simulink model "Cruise_model"  (R2020a)
settings: Solver=ode15s  StartTime=0.0  StopTime=30  MaxStep=0.1  RelTol=1e-3
values from neighbouring files (symbols this model uses):
  b = 50    [Initialization.mat]
  m = 1000    [Initialization.mat]
settings Model: DataDictionary=Ques_3_Parameters.sldd  Creator=DELL  LastModifiedBy=DELL

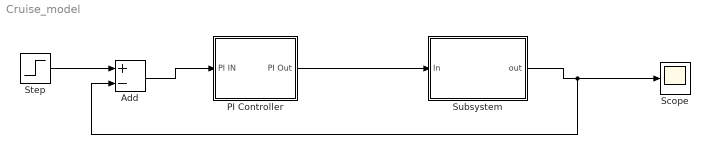
== system Cruise_model ==
  Add : Sum  Inputs=+-
  PI Controller : Subsystem
  Scope : Scope
  Step : Step  After=u  SampleTime=0
  Subsystem : Subsystem
  wires:
  Subsystem/1(out) -> Add/2, Scope/1
  PI Controller/1(PI Out) -> Subsystem/1(In)
  Step/1 -> Add/1
  Add/1 -> PI Controller/1(PI IN)

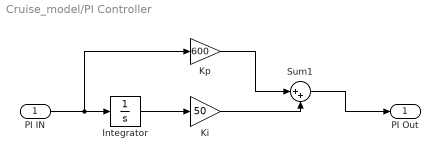
== system Cruise_model/PI Controller ==
  PI IN : Inport  OutDataTypeStr=double  PortDimensions=1  SampleTime=0
  Integrator : Integrator
  Ki : Gain  Gain=50
  Kp : Gain  Gain=600
  Sum1 : Sum  Inputs=|++
  PI Out : Outport  OutDataTypeStr=double  PortDimensions=1  SampleTime=0
  wires:
  Ki/1 -> Sum1/2
  PI IN/1 -> Integrator/1, Kp/1
  Kp/1 -> Sum1/1
  Sum1/1 -> PI Out/1
  Integrator/1 -> Ki/1

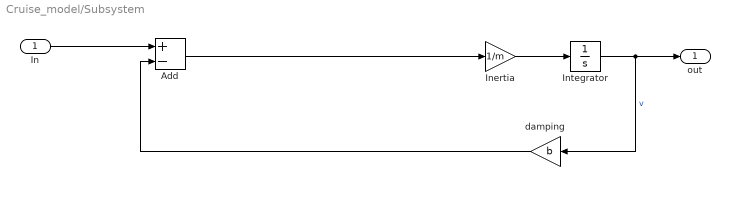
== system Cruise_model/Subsystem ==
  In : Inport
  Add : Sum  Inputs=+-
  Inertia : Gain  Gain=1/m
  Integrator : Integrator
  damping : Gain  Gain=b
  out : Outport
  wires:
  In/1 -> Add/1
  damping/1 -> Add/2
  Integrator/1 -> out/1, damping/1  "v"
  Inertia/1 -> Integrator/1
  Add/1 -> Inertia/1
